simulink model "updated_target_driver_2026_withVariants_MPC_andwlqp2"  (R2024b)
settings: Solver=FixedStepDiscrete  StartTime=0.0  StopTime=running_time  FixedStep=dt_s  RelTol=1e-3
values from neighbouring files (symbols this model uses):
  A = gamma_2*gamma_3*Thrust_desired    [force2voltage.m]
  a2_lb = -0.25    [target_driver_setup_2022_Ctrl_V_2_4.m]    (also in target_driver_setup_2022_Ctrl_V_2_4_geometric.m; target_driver_setup_mpc_12msdelay.m; target_driver_setup_mpc_andWLQP.m)
  a2_openloop = -0    (= 0)    [target_driver_setup_2022_Ctrl_V_2_4.m]    (also in target_driver_setup_2022_Ctrl_V_2_4_geometric.m; target_driver_setup_mpc_12msdelay.m; target_driver_setup_mpc_andWLQP.m)
  a2_ub = 0.25    [target_driver_setup_2022_Ctrl_V_2_4.m]    (also in target_driver_setup_2022_Ctrl_V_2_4_geometric.m; target_driver_setup_mpc_12msdelay.m; target_driver_setup_mpc_andWLQP.m)
  att_s = 500    [target_driver_setup_2022_Ctrl_V_2_4.m]    (also in target_driver_setup_2022_Ctrl_V_2_4_geometric.m; target_driver_setup_mpc_12msdelay.m; target_driver_setup_mpc_andWLQP.m)
  c_vertical = 0.70e-3    (= 0.0007)    [target_driver_setup_mpc_andWLQP.m]
  closedloop_flag = 1    [target_driver_setup_2022_Ctrl_V_2_4.m]    (also in target_driver_setup_2022_Ctrl_V_2_4_geometric.m = 0; target_driver_setup_mpc_12msdelay.m = 0; target_driver_setup_mpc_andWLQP.m = 0)
  delay = delay-vicon_sample_cycle/2    [target_driver_setup_2022_Ctrl_V_2_4.m]    (also in target_driver_setup_2022_Ctrl_V_2_4_geometric.m; target_driver_setup_mpc_12msdelay.m; target_driver_setup_mpc_andWLQP.m)
  drv_amp = abs((vleft_p2p-vright_p2p))/2+min(vleft_p2p,vright_p2p)    [Wing_traj_to_Voltage.m]    (also in force2voltage.m; target_driver_setup_2022_Ctrl_V_2_4.m = 300; target_driver_setup_2022_Ctrl_V_2_4_geometric.m = 110; target_driver_setup_mpc_12msdelay.m = 150)
  drv_bias = max_drv_bias    (= 300)    [target_driver_setup_2022_Ctrl_V_2_4.m]    (also in target_driver_setup_2022_Ctrl_V_2_4_geometric.m = 200; target_driver_setup_mpc_12msdelay.m = 200; target_driver_setup_mpc_andWLQP.m = 200)
  drv_pitch_left = vleft_pitch    [Wing_traj_to_Voltage.m]    (also in force2voltage.m = 0; target_driver_setup_2022_Ctrl_V_2_4.m = 0; target_driver_setup_2022_Ctrl_V_2_4_geometric.m = 9.05; target_driver_setup_mpc_12msdelay.m = 9.05)
  drv_pitch_right = vright_pitch    [Wing_traj_to_Voltage.m]    (also in force2voltage.m = 0; target_driver_setup_2022_Ctrl_V_2_4.m = 0; target_driver_setup_2022_Ctrl_V_2_4_geometric.m = 9.05; target_driver_setup_mpc_12msdelay.m = 9.05)
  drv_roll = (vleft_p2p-vright_p2p)/4    [Wing_traj_to_Voltage.m]    (also in force2voltage.m; target_driver_setup_2022_Ctrl_V_2_4.m = 0; target_driver_setup_2022_Ctrl_V_2_4_geometric.m = -0.001; target_driver_setup_mpc_12msdelay.m = -0.001)
  dt_s = 1e-3    (= 0.001)    [target_driver_setup_2022_Ctrl_V_2_4.m]    (also in target_driver_setup_2022_Ctrl_V_2_4_geometric.m = 0.0002; target_driver_setup_mpc_12msdelay.m = 0.0002; target_driver_setup_mpc_andWLQP.m = 2.0e-4;1)
  f_fin = f    (= 180)    [target_driver_setup_2022_Ctrl_V_2_4.m]    (also in target_driver_setup_2022_Ctrl_V_2_4_geometric.m = 155; target_driver_setup_mpc_12msdelay.m = 155; target_driver_setup_mpc_andWLQP.m = 155)
  f_int = f    (= 180)    [target_driver_setup_2022_Ctrl_V_2_4.m]    (also in target_driver_setup_2022_Ctrl_V_2_4_geometric.m = 155; target_driver_setup_mpc_12msdelay.m = 155; target_driver_setup_mpc_andWLQP.m = 155)
  g = 9.8    [target_driver_setup_2022_Ctrl_V_2_4.m]    (also in target_driver_setup_2022_Ctrl_V_2_4_geometric.m; target_driver_setup_mpc_12msdelay.m; target_driver_setup_mpc_andWLQP.m = 9.81; test_full_attitude_mpc.m = 9.81)
  I_moment = eye(3)    [target_driver_exec_2022_Ctrl_V_2_4.m]    (also in target_driver_setup_2022_Ctrl_V_2_4.m; target_driver_setup_2022_Ctrl_V_2_4_geometric.m; target_driver_setup_mpc_12msdelay.m; target_driver_setup_mpc_andWLQP.m)
  k_tau_vec = [k_tau_roll;k_tau_pitch]    [target_driver_setup_2022_Ctrl_V_2_4_geometric.m]    (also in target_driver_setup_mpc_12msdelay.m; target_driver_setup_mpc_andWLQP.m)
  m = t <= t_zoom    [plot_roll_torque_cmd_vs_actual.m]    (also in plot_roll_torque_cmd_vs_actual_flightlog.m = t >= t0 & t <= t1; target_driver_setup_2022_Ctrl_V_2_4.m = 0.000124; target_driver_setup_2022_Ctrl_V_2_4_geometric.m = 8.5655e-05; target_driver_setup_mpc_12msdelay.m = 8.5655e-05)
  params_vec = [params_opt.delta_1, params_opt.delta_2, params_opt.delta_3,      params_opt.gamma_1, params_opt.gamma_2_1, params_opt.gamma_3,      params_opt.eta, params_opt.nu, params_opt.mu]'    [force2voltage_tuningSandbox.m]    (also in target_driver_setup_2022_Ctrl_V_2_4.m = [params_opt.delta_1, params_opt.delta_2, params_opt.delta_3,; target_driver_setup_2022_Ctrl_V_2_4_geometric.m = [params_opt.delta_1, params_opt.delta_2, params_opt.delta_3,; target_driver_setup_mpc_12msdelay.m = [params_opt.delta_1, params_opt.delta_2, params_opt.delta_3,; target_driver_setup_mpc_andWLQP.m = [params_opt.delta_1, params_opt.delta_2, params_opt.delta_3,)
  phase = 0    [target_driver_setup_2022_Ctrl_V_2_4.m]    (also in target_driver_setup_2022_Ctrl_V_2_4_geometric.m; target_driver_setup_mpc_12msdelay.m; target_driver_setup_mpc_andWLQP.m)
  popts_flattened = popts.popts    [target_driver_setup_mpc_andWLQP.m]
  roll_offset_angle = 0    [target_driver_setup_2022_Ctrl_V_2_4.m]    (also in target_driver_setup_2022_Ctrl_V_2_4_geometric.m; target_driver_setup_mpc_12msdelay.m; target_driver_setup_mpc_andWLQP.m)
  running_time = start_delay+total_T    (= 9)    [target_driver_setup_2022_Ctrl_V_2_4.m]    (also in target_driver_setup_2022_Ctrl_V_2_4_geometric.m = 10; target_driver_setup_mpc_12msdelay.m = 0.5; target_driver_setup_mpc_andWLQP.m = 10)
  running_time_control = start_delay_control+total_T+0.0    (= 7.1)    [target_driver_setup_2022_Ctrl_V_2_4.m]    (also in target_driver_setup_2022_Ctrl_V_2_4_geometric.m = 10; target_driver_setup_mpc_12msdelay.m = 0.5; target_driver_setup_mpc_andWLQP.m = 10)
  sampling_f = 10000    [target_driver_setup_2022_Ctrl_V_2_4.m]    (also in target_driver_setup_2022_Ctrl_V_2_4_geometric.m = 5000; target_driver_setup_mpc_12msdelay.m = 5000; target_driver_setup_mpc_andWLQP.m = 1/dt_s)
  start_delay = 2.0    (= 2)    [target_driver_setup_2022_Ctrl_V_2_4.m]    (also in target_driver_setup_2022_Ctrl_V_2_4_geometric.m = 0; target_driver_setup_mpc_12msdelay.m = 0; target_driver_setup_mpc_andWLQP.m = 0)
  start_delay_control = start_delay + ramp_delay    (= 0.1)    [target_driver_setup_2022_Ctrl_V_2_4.m]    (also in target_driver_setup_2022_Ctrl_V_2_4_geometric.m = 0; target_driver_setup_mpc_12msdelay.m = 0; target_driver_setup_mpc_andWLQP.m = 0)
  T = 1    [target_driver_setup_2022_Ctrl_V_2_4.m]    (also in target_driver_setup_2022_Ctrl_V_2_4_geometric.m = 10; target_driver_setup_mpc_12msdelay.m = 0.5; target_driver_setup_mpc_andWLQP.m = 10; test_full_attitude_mpc.m = T0 + nu(1))
  weights_vec = [ws; wds; wpr_xy;wpr_z; wpf; wvr_xy; wvr_z ... (first row only)    [target_driver_setup_2022_Ctrl_V_2_4_geometric.m]    (also in target_driver_setup_mpc_12msdelay.m; target_driver_setup_mpc_andWLQP.m)
undefined symbols (not defined in the file or in its folder): Com1, ctrl_Ts, DiscIntNeverNeededParam, dspblkCoreblockFVToolHelper, gcbh, left_mapping, left_mapping_F_to_Phi, lp_den, lp_num, none, right_mapping, right_mapping_F_to_Phi
libraries: simulink x17, xpcseriallib x2, cstblocks x1, xpcnilib x1, xpcutilitieslib x1
(part 1 of 4)
settings Model: PacingRate=0.020000  Creator=franklinho  LastModifiedBy=franklinho
settings DebuggingCC: SignalInfNanChecking=error  UnderSpecifiedDimensionMsg=warning

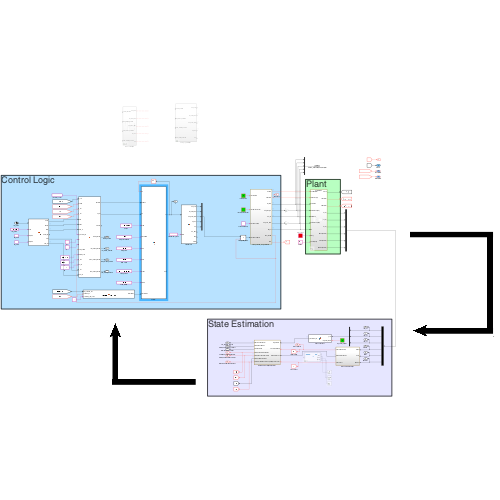
[thumbnail: Simulink's stored preview of the top-level diagram]
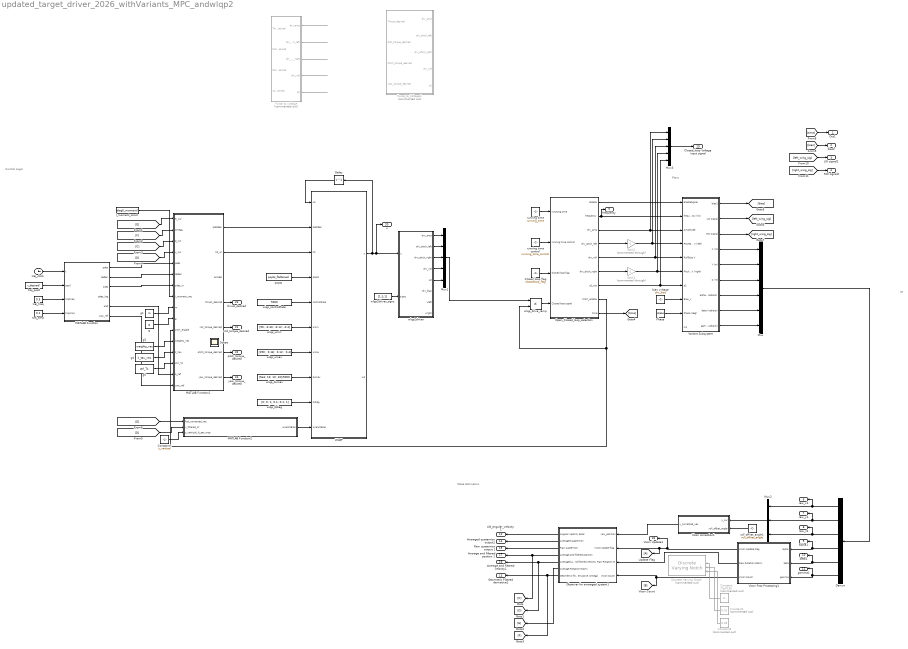
== system updated_target_driver_2026_withVariants_MPC_andwlqp2 ==
  note: te
  note: Plant
  note: State Estimation
  note: Control Logic
  Closed loop flag : Constant  Value=closedloop_flag
  Constant : Constant  Commented=on  Value=2*pi*155
  Constant1 : Constant  Commented=on  Value=0.01
  Constant2 : Constant  Commented=on  Value=0.05
  Constant3 : Constant  Value=c_vertical
  Delay : Delay  DelayLength=1  InitialCondition=[120; 0; 0; 0]
  Demux : Demux  Outputs=6
  Discrete Varying Notch : cstblocks/Linear Parameter Varying/Discrete Varying Notch  Commented=on  w0=973.894  Ts=2e-4
  Force to voltage : Subsystem  Commented=on  Variant=on
  Force_to_Voltage1 : Subsystem  Commented=on
  Gain2 : Gain  Commented=through  Gain=-1
  Gain3 : Gain  Commented=through  Gain=-1
  I_moment_const : Constant  Value=diag(I_moment)
  MATLAB Function : MATLAB Function  TreatAsAtomicUnit=on
  MATLAB Function1 : MATLAB Function  TreatAsAtomicUnit=on
  MATLAB Function2 : MATLAB Function  TreatAsAtomicUnit=on
  Mux : Mux  Inputs=6
  Mux1 : Mux  Inputs=5
  Mux2 : Mux  Inputs=3
  Mux3 : Mux  Inputs=5
  Observer for averaged system1 : Subsystem
  Open_Closed_loop_selection : Subsystem
  Phase : Constant  Value=phase
  Update Flag : Goto
  Variant Subsystem : Subsystem  Variant=on
  Vicon Post Processing1 : Subsystem
  Vicon correction1 : MATLAB Function  TreatAsAtomicUnit=on
  WLQP : MATLAB Function  TreatAsAtomicUnit=on
  bias voltage : Constant  Value=drv_bias
  g : Constant  Value=g
  g1 : Constant  Value=m
  g3 : Constant  Value=weights_vec
  g4 : Constant  Value=k_tau_vec
  g5 : Constant  Value=ctrl_Ts
  popts : Constant  Value=popts_flattened
  roll_offset_angle1 : Constant  Value=roll_offset_angle  SampleTime=-1
  running time : Constant  Value=running_time  SampleTime=-1
  running time control : Constant  Value=running_time_control  SampleTime=-1
  traj_amp : Constant  Value=0.1
  traj_clock : Clock
  traj_freq : Constant  Value=0.5
  traj_pos0 : Constant  Value=r_desired'
  wlqp2driver : MATLAB Function  TreatAsAtomicUnit=on
  wlqp2driver_signs : Constant  Value=[1;1;1]
  wlqp_Qdiag : Constant  Value=[0; 0; 1; 0.1; 0.1; 1]
  wlqp_controlRate : Constant  Value=5000
  wlqp_drive_ramp : Product
  wlqp_dumax : Constant  Value=[5e3; 10; 10; 10]/5000
  wlqp_umax : Constant  Value="[190;  0.18;  0.12;  0.4]"
  wlqp_umin : Constant  Value=[90; -0.40; -0.12; -0.4]
  Out1 : Outport
  bias2 : Outport  Port=2
  LW signal2 : Outport  Port=3
  RW signal2 : Outport  Port=4
  frequency : Outport  Port=5
  raw_x1 : Outport  Port=6
  raw_y1 : Outport  Port=7
  raw_z1 : Outport  Port=8
  alpha1 : Outport  Port=9
  beta1 : Outport  Port=10
  gamma1 : Outport  Port=11
  old_angular_velocity 1 : Outport  Port=12
  Geometric Filtered derivative1 : Outport  Port=13
  Averaged quaternion output1 : Outport  Port=14
  Raw quaternion output 1 : Outport  Port=15
  Average and filtered velocity1 : Outport  Port=16
  Average and filtered position 1 : Outport  Port=17
  Vicon Update1 : Outport  Port=18
  Closed_loop Voltage input signal : Outport  Port=19
  u : Outport  Port=20
  roll_torque_desired : Outport  Port=21
  pitch_torque_desired : Outport  Port=22
  thrust_desired : Outport  Port=23
  yaw_torque_desired : Outport  Port=24
  Scope : Scope
  wires:
  Observer for averaged system1/1("Angular velocity Euler ") -> old_angular_velocity 1/1
  Observer for averaged system1/5(Averaged and filtered velocity) -> [D], Average and filtered velocity1/1
  Observer for averaged system1/2(Averaged quaternion) -> Averaged quaternion output1/1
  roll_offset_angle1/1 -> Vicon correction1/2(roll_offset_angle)
  Observer for averaged system1/4("Average and filtered position ") -> Average and filtered position 1/1, [C]
  Observer for averaged system1/3(Raw quaternion) -> Raw quaternion output 1/1
  Vicon Post Processing1/1("Vicon Update Flag ") -> Vicon Update1/1, Update Flag/1, Observer for averaged system1/2(Vicon Update flag)
  Observer for averaged system1/7(Geometric filtered derivative (omega)) -> [F], Geometric Filtered derivative1/1
  Mux2/1 -> Vicon correction1/1(x_cur)
  Vicon Post Processing1/3("Vicon Count ") -> Observer for averaged system1/4(Vicon Count), [B]
  Vicon correction1/1(x_corrected_vec) -> Observer for averaged system1/1("raw_position ")
  Variant Subsystem/4(X (m)) -> Mux/1
  Variant Subsystem/5(Y (m)) -> Mux/2
  Variant Subsystem/6(Z (m)) -> Mux/3
  Variant Subsystem/7(alpha (radians)) -> Mux/4
  Variant Subsystem/8(beta (radians)) -> Mux/5
  Variant Subsystem/9(gamma (radians)) -> Mux/6
  Variant Subsystem/1(bias2) -> [bias]
  Variant Subsystem/2(LW signal) -> [left_wing_sig]
  Variant Subsystem/3(RW signal) -> [right_wing_sig]
  Mux/1 -> Demux/1
  Demux/1 -> raw_x1/1, Mux2/1
  Demux/3 -> raw_z1/1, Mux2/3
  Demux/2 -> raw_y1/1, Mux2/2
  Demux/4 -> alpha1/1, Vicon Post Processing1/1(alpha)
  Demux/5 -> beta1/1, Vicon Post Processing1/2(beta)
  Demux/6 -> gamma1/1, Vicon Post Processing1/3(gamma)
  running time control/1 -> Open_Closed_loop_selection/2("running time control ")
  Closed loop flag/1 -> Open_Closed_loop_selection/3(Closed loop flag)
  running time/1 -> Open_Closed_loop_selection/1(runnting time)
  Open_Closed_loop_selection/1("Enable ") -> Variant Subsystem/1(EnableSignal)
  Open_Closed_loop_selection/2(frequency) -> Variant Subsystem/2(frequency (hz)), frequency/1
  Open_Closed_loop_selection/3(drv_amp) -> Mux3/1, Variant Subsystem/3(Amplitude)
  Open_Closed_loop_selection/4("drv_pitch_left ") -> Gain2/1
  Open_Closed_loop_selection/6("drv_pitch_right ") -> Gain3/1
  Open_Closed_loop_selection/7(a2_out) -> Mux3/5, Variant Subsystem/7(a2)
  Open_Closed_loop_selection/9(time) -> [time]
  bias voltage/1 -> Variant Subsystem/8(Bias_v)
  Phase/1 -> Variant Subsystem/9(Phase (deg))
  Mux3/1 -> Closed_loop Voltage input signal/1
  [time] -> Out1/1
  [bias] -> bias2/1
  [left_wing_sig] -> LW signal2/1
  [right_wing_sig] -> RW signal2/1
  Open_Closed_loop_selection/5("drv_roll ") -> Mux3/3, Variant Subsystem/5(RollBias V)
  Vicon Post Processing1/2(Raw Rotation Matrix) -> Observer for averaged system1/3("Raw Rotation M ")
  Constant/1 -> Discrete Varying Notch/2
  Constant1/1 -> Discrete Varying Notch/3
  Constant2/1 -> Discrete Varying Notch/4
  Gain2/1 -> Mux3/2, Variant Subsystem/4(PitchBias V (left))
  Gain3/1 -> Mux3/4, Variant Subsystem/6(PitchBias V (right))
  g/1 -> MATLAB Function1/10(g)
  g1/1 -> MATLAB Function1/9(m)
  MATLAB Function/1(pdes) -> MATLAB Function1/5(pdes)
  MATLAB Function/2(dpdes) -> MATLAB Function1/6(dpdes)
  MATLAB Function/3(sdes) -> MATLAB Function1/7(sdes_in)
  [E] -> MATLAB Function1/1(R_cur)
  [F] -> MATLAB Function1/2(omega)
  Open_Closed_loop_selection/8(Cntrl_enable) -> wlqp_drive_ramp/2, MATLAB Function1/11(cntrl_enable)
  g3/1 -> MATLAB Function1/12(weights_vec)
  g4/1 -> MATLAB Function1/13(k_tau)
  g5/1 -> MATLAB Function1/14(ctrl_Ts)
  [C] -> MATLAB Function1/3(p_cur)
  [D] -> MATLAB Function1/4(v_cur)
  WLQP/1(u) -> u/1, wlqp2driver/1(u), Delay/1
  Delay/1 -> WLQP/1(u0)
  MATLAB Function1/2(h0_wl) -> WLQP/3(h0)
  MATLAB Function1/1(pdotdes) -> WLQP/2(pdotdes)
  Force to voltage/2(drv_pitch_left) -> ?
  Force to voltage/4(drv_roll) -> ?
  Force to voltage/5(a2) -> ?
  Force to voltage/3(drv_pitch_right) -> ?
  Force to voltage/1(drv_amp) -> ?
  wlqp2driver/1(drv_amp) -> Mux1/1
  wlqp2driver/2(drv_pitch_left) -> Mux1/2
  wlqp2driver/3(drv_pitch_right) -> Mux1/3
  wlqp2driver/4(drv_roll) -> Mux1/4
  wlqp2driver/5(a2) -> Mux1/5
  popts/1 -> WLQP/4(popts)
  traj_clock/1 -> MATLAB Function/1(t)
  traj_pos0/1 -> MATLAB Function/2(pos0)
  traj_freq/1 -> MATLAB Function/3(trajFreq)
  traj_amp/1 -> MATLAB Function/4(trajAmp)
  I_moment_const/1 -> MATLAB Function1/8(I_moment_vec)
  wlqp_controlRate/1 -> WLQP/5(controlRate)
  wlqp_umin/1 -> WLQP/6(umin)
  wlqp_umax/1 -> WLQP/7(umax)
  wlqp_dumax/1 -> WLQP/8(dumax)
  wlqp_Qdiag/1 -> WLQP/9(Qdiag)
  MATLAB Function1/5(roll_torque_desired) -> roll_torque_desired/1
  MATLAB Function1/6(pitch_torque_desired) -> pitch_torque_desired/1
  wlqp2driver_signs/1 -> wlqp2driver/2(signs)
  MATLAB Function1/4(thrust_desired) -> thrust_desired/1
  Mux1/1 -> wlqp_drive_ramp/1
  wlqp_drive_ramp/1 -> Open_Closed_loop_selection/4(Closed loop signal)
  MATLAB Function/5(aref) -> MATLAB Function1/15(a_ref)
  MATLAB Function1/7(yaw_torque_desired) -> yaw_torque_desired/1
  Observer for averaged system1/6(Average Rotation Matrix) -> [E]
  MATLAB Function2/1(wrenchBias) -> WLQP/10(wrenchBias)
  [D] -> MATLAB Function2/2(v_filtered_W)
  Constant3/1 -> MATLAB Function2/3(c_vertical_N_per_mps)
  [E] -> MATLAB Function2/1(Rot_corrected_vec)
  MATLAB Function/6(yaw_ref) -> MATLAB Function1/16(yaw_ref)

== system updated_target_driver_2026_withVariants_MPC_andwlqp2/Force to voltage ==
  note: 1) Add Subsystem or Model blocks as valid variant choices.
      | 2) You cannot connect blocks at this level. At simulation, connectivity is automatically
      | determined, based on the active variant and port name matching.
  "Thrust_desired " : Inport
  Roll_torque_desired : Inport  Port=2
  Pitch_torque_desired : Inport  Port=3
  Yaw_torque_desired : Inport  Port=4
  Control Mode : Subsystem  VariantControl=replay_mode==1
  Replay Mode : Subsystem  VariantControl=replay_mode==2
  drv_amp : Outport
  drv_pitch_left : Outport  Port=2
  drv_pitch_right : Outport  Port=3
  drv_roll : Outport  Port=4
  a2 : Outport  Port=5

== system updated_target_driver_2026_withVariants_MPC_andwlqp2/Force_to_Voltage1 ==
  note: Mapping from desired Thrust/Torque to Wing traj to Voltage mapping
      |
      | Patrick Hyun 2021 Apr
  note: a2: second-harmonic coefficient
      | Franklin Ho Jun 2026
  "Thrust_desired " : Inport
  Roll_torque_desired : Inport  Port=2
  Pitch_torque_desired : Inport  Port=3
  Yaw_torque_desired : Inport  Port=4
  A : Constant  Commented=on  Value=A
  Desired_Force_to_Voltage : MATLAB Function  TreatAsAtomicUnit=on
  "Force to Trajectory " : MATLAB Function  Commented=on  TreatAsAtomicUnit=on
  Saturation : Saturate  UpperLimit=a2_ub  LowerLimit=a2_lb
  "Trajectory to Voltage Input " : MATLAB Function  Commented=on  TreatAsAtomicUnit=on
  left_mapping : Constant  Commented=on  Value=left_mapping
  left_mapping_F_to_Phi : Constant  Commented=on  Value=left_mapping_F_to_Phi
  params_vec : Constant  Value=params_vec
  right_mapping1 : Constant  Commented=on  Value=right_mapping
  right_mapping_F_to_Phi : Constant  Commented=on  Value=right_mapping_F_to_Phi
  drv_amp : Outport
  drv_pitch_left : Outport  Port=2
  drv_pitch_right : Outport  Port=3
  drv_roll : Outport  Port=4
  a2 : Outport  Port=5
  wires:
  left_mapping/1 -> "Trajectory to Voltage Input "/4(left_mapping)
  right_mapping1/1 -> "Trajectory to Voltage Input "/5(right_mapping)
  A/1 -> "Force to Trajectory "/6(A)
  "Force to Trajectory "/1(Phi_left_p2p_desired) -> "Trajectory to Voltage Input "/1(Phi_left_p2p_command)
  "Force to Trajectory "/2(Phi_right_p2p_desired) -> "Trajectory to Voltage Input "/2(Phi_right_p2p_command)
  "Force to Trajectory "/3(Phi_pitch_desired) -> "Trajectory to Voltage Input "/3(Phi_pitch_command)
  left_mapping_F_to_Phi/1 -> "Force to Trajectory "/4(left_mapping_F_to_Phi)
  right_mapping_F_to_Phi/1 -> "Force to Trajectory "/5(right_mapping_F_to_Phi)
  Desired_Force_to_Voltage/4(drv_pitch_right) -> drv_pitch_right/1
  Desired_Force_to_Voltage/3(drv_pitch_left) -> drv_pitch_left/1
  Desired_Force_to_Voltage/2(drv_roll) -> drv_roll/1
  Desired_Force_to_Voltage/1(drv_amp) -> drv_amp/1
  "Thrust_desired "/1 -> Desired_Force_to_Voltage/1(Thrust_desired)
  Pitch_torque_desired/1 -> Desired_Force_to_Voltage/3(Pitch_torque_desired)
  Yaw_torque_desired/1 -> Desired_Force_to_Voltage/4(Yaw_torque_desired)
  params_vec/1 -> Desired_Force_to_Voltage/5(params_vec)
  Desired_Force_to_Voltage/5(a2_coeff) -> Saturation/1
  Saturation/1 -> a2/1
  Roll_torque_desired/1 -> Desired_Force_to_Voltage/2(Roll_torque_desired)

== system updated_target_driver_2026_withVariants_MPC_andwlqp2/Observer for averaged system1 ==
  note: Observer for averaged system using geoemtric average
      | Includes the Euler derivatives to compute the angular velocity (probably not used for control)
      | Includes the geometric average and the first order derivative in Riemannian metric SO(3)
      |
      | Patrick 2021 Mar
  "raw_position " : Inport
  Vicon Update flag : Inport  Port=2
  "Raw Rotation M " : Inport  Port=3
  Vicon Count : Inport  Port=4
  Attitude Observer : Subsystem
  "Euler derivative & filtered angular velocity " : Subsystem
  Position Observer : Subsystem
  Terminator : Terminator
  "Angular velocity Euler " : Outport
  Averaged quaternion : Outport  Port=2
  Raw quaternion : Outport  Port=3
  "Average and filtered position " : Outport  Port=4
  Averaged and filtered velocity : Outport  Port=5
  Average Rotation Matrix : Outport  Port=6
  Geometric filtered derivative (omega) : Outport  Port=7
  wires:
  "Raw Rotation M "/1 -> "Euler derivative & filtered angular velocity "/1("Rotation matrix "), Attitude Observer/2(Raw Rotation)
  Vicon Count/1 -> Attitude Observer/3(Vicon Count), Position Observer/3(Vicon Count)
  "raw_position "/1 -> Position Observer/1("raw_position ")
  Position Observer/1(Average and filtered position) -> "Average and filtered position "/1
  Position Observer/2(Averaged and filtered velocity) -> Averaged and filtered velocity/1
  "Euler derivative & filtered angular velocity "/1(Angular velocity_Euler) -> "Angular velocity Euler "/1
  Vicon Update flag/1 -> Attitude Observer/1(Vicon Update flag), Position Observer/2(vicon Update)
  Attitude Observer/1("Averaged quaternion ") -> Averaged quaternion/1
  Attitude Observer/2(Average Rotation Matrix) -> Average Rotation Matrix/1
  Attitude Observer/3(Raw quaternion) -> Raw quaternion/1
  Attitude Observer/4(Geometric filtered derivative) -> Geometric filtered derivative (omega)/1
  "Euler derivative & filtered angular velocity "/2(Frob_norm error) -> Terminator/1

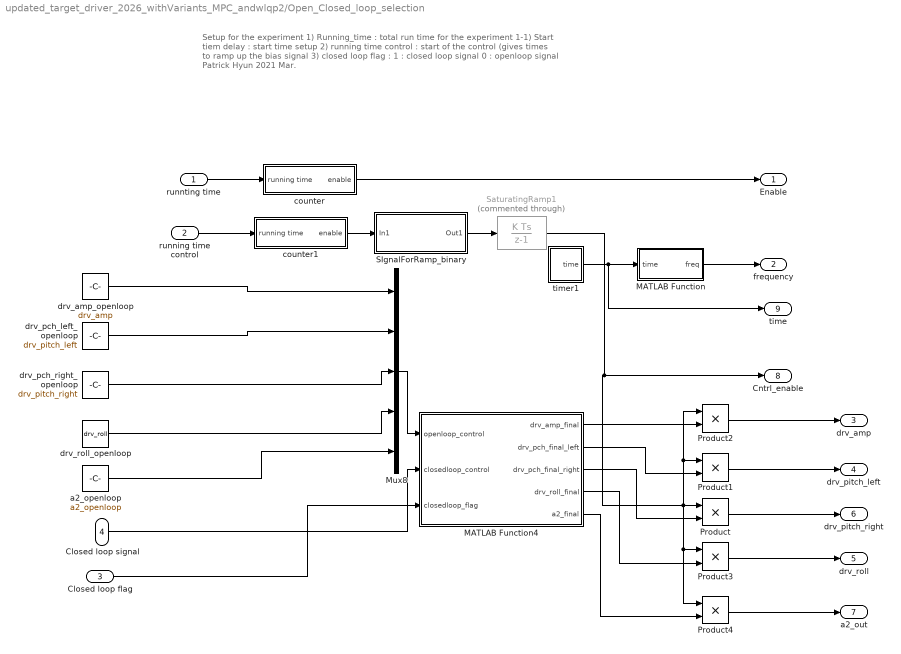
== system updated_target_driver_2026_withVariants_MPC_andwlqp2/Open_Closed_loop_selection ==
  note: Setup for the experiment
      |
      | 1) Running_time : total run time for the experiment
      | 1-1) Start tiem delay : start time setup
      | 2) running time control : start of the control (gives times to ramp up the bias signal
      | 3) closed loop flag : 1 : closed loop signal 0 : openloop signal
      |
      | Patrick Hyun 2021 Mar.
  runnting time : Inport
  "running time control " : Inport  Port=2
  Closed loop flag : Inport  Port=3
  Closed loop signal : Inport  Port=4
  MATLAB Function : MATLAB Function  TreatAsAtomicUnit=on
  MATLAB Function4 : MATLAB Function  TreatAsAtomicUnit=on
  Mux8 : Mux  Inputs=5
  Product{,1..4} (5 alike) : Product  RndMeth=Zero
  SIgnalForRamp_binary : Subsystem
  SaturatingRamp1 : DiscreteIntegrator  Commented=through  gainval=2.5  SampleTime=-1  LimitOutput=on  UpperSaturationLimit=1  LowerSaturationLimit=0  ICPrevOutput=DiscIntNeverNeededParam  ICPrevScaledInput=DiscIntNeverNeededParam
  a2_openloop : Constant  Value=a2_openloop
  counter : Subsystem
  counter1 : Subsystem
  "drv_amp_openloop " : Constant  Value=drv_amp
  drv_pch_left_openloop : Constant  Value=drv_pitch_left
  drv_pch_right_openloop : Constant  Value=drv_pitch_right
  "drv_roll_openloop " : Constant  Value=drv_roll
  timer1 : Subsystem
  "Enable " : Outport
  frequency : Outport  Port=2
  drv_amp : Outport  Port=3
  "drv_pitch_left " : Outport  Port=4
  "drv_roll " : Outport  Port=5
  "drv_pitch_right " : Outport  Port=6
  a2_out : Outport  Port=7
  Cntrl_enable : Outport  Port=8
  time : Outport  Port=9
  wires:
  runnting time/1 -> counter/1(running time)
  timer1/1(time) -> time/1, MATLAB Function/1(time)
  MATLAB Function/1(freq) -> frequency/1
  SIgnalForRamp_binary/1(Out1) -> SaturatingRamp1/1
  "drv_amp_openloop "/1 -> Mux8/1
  Product1/1 -> "drv_pitch_left "/1
  counter1/1(enable) -> SIgnalForRamp_binary/1(In1)
  "running time control "/1 -> counter1/1(running time)
  Product3/1 -> "drv_roll "/1
  Closed loop flag/1 -> MATLAB Function4/3(closedloop_flag)
  MATLAB Function4/4(drv_roll_final) -> Product3/2
  Mux8/1 -> MATLAB Function4/1(openloop_control)
  MATLAB Function4/2(drv_pch_final_left) -> Product1/2
  Product2/1 -> drv_amp/1
  MATLAB Function4/1(drv_amp_final) -> Product2/2
  drv_pch_left_openloop/1 -> Mux8/2
  MATLAB Function4/3(drv_pch_final_right) -> Product/2
  Product/1 -> "drv_pitch_right "/1
  counter/1(enable) -> "Enable "/1
  Closed loop signal/1 -> MATLAB Function4/2(closedloop_control)
  "drv_roll_openloop "/1 -> Mux8/4
  drv_pch_right_openloop/1 -> Mux8/3
  Product4/1 -> a2_out/1
  MATLAB Function4/5(a2_final) -> Product4/2
  a2_openloop/1 -> Mux8/5
  SaturatingRamp1/1 -> Product4/1, Product3/1, Product2/1, Product1/1, Product/1, Cntrl_enable/1

== system updated_target_driver_2026_withVariants_MPC_andwlqp2/Variant Subsystem ==
  note: 1) Add Subsystem or Model blocks as valid variant choices.
      | 2) You cannot connect blocks at this level. At simulation, connectivity is automatically
      | determined, based on the active variant and port name matching.
  EnableSignal : Inport
  frequency (hz) : Inport  Port=2
  Amplitude : Inport  Port=3
  PitchBias V (left) : Inport  Port=4
  RollBias V : Inport  Port=5
  PitchBias V (right) : Inport  Port=6
  a2 : Inport  Port=7
  Bias_v : Inport  Port=8
  Phase (deg) : Inport  Port=9
  In1 : Inport  Port=10
  Experimental : Subsystem  VariantControl=Plant==1
  Simulation : Subsystem  VariantControl=Plant==2
  bias2 : Outport
  LW signal : Outport  Port=2
  RW signal : Outport  Port=3
  X (m) : Outport  Port=4
  Y (m) : Outport  Port=5
  Z (m) : Outport  Port=6
  alpha (radians) : Outport  Port=7
  beta (radians) : Outport  Port=8
  gamma (radians) : Outport  Port=9

== system updated_target_driver_2026_withVariants_MPC_andwlqp2/Vicon Post Processing1 ==
  note: Process Vicon data
      |
      | 1) Generate Raw rotation matrix
      | 2) Flag the update of new vicon data
      | 3) Count the number of samples before new update
      |
      | By Patrick 2021 Mar
  alpha : Inport
  beta : Inport  Port=2
  gamma : Inport  Port=3
  Raw rotation matrix : Subsystem
  Vicon Validity check : Subsystem
  Vicon correction : MATLAB Function  TreatAsAtomicUnit=on
  roll_offset_angle : Constant  Value=roll_offset_angle  SampleTime=-1
  "Vicon Update Flag " : Outport
  Raw Rotation Matrix : Outport  Port=2
  "Vicon Count " : Outport  Port=3
  wires:
  Vicon Validity check/2(Vicon Count) -> "Vicon Count "/1
  beta/1 -> Raw rotation matrix/2(beta)
  gamma/1 -> Raw rotation matrix/3(gamma)
  alpha/1 -> Raw rotation matrix/1(alpha)
  Vicon Validity check/1("Vicon Update flag ") -> "Vicon Update Flag "/1
  roll_offset_angle/1 -> Vicon correction/2(roll_offset_angle)
  Raw rotation matrix/1(R) -> Vicon correction/1(R_cur)
  Vicon correction/1(Rot_corrected_vec) -> Raw Rotation Matrix/1, Vicon Validity check/1("Rotation Matrix ")

== system updated_target_driver_2026_withVariants_MPC_andwlqp2/Force to voltage/Control Mode ==
  "Thrust_desired " : Inport
  Roll_torque_desired : Inport  Port=2
  Pitch_torque_desired : Inport  Port=3
  Yaw_torque_desired : Inport  Port=4
  Desired_Force_to_Voltage : MATLAB Function  TreatAsAtomicUnit=on
  Force_to_Voltage1 : Subsystem  Commented=on
  Saturation : Saturate  UpperLimit=a2_ub  LowerLimit=a2_lb
  params_vec : Constant  Value=params_vec
  drv_amp : Outport
  drv_pitch_left : Outport  Port=2
  drv_pitch_right : Outport  Port=3
  drv_roll : Outport  Port=4
  a2 : Outport  Port=5
  wires:
  Desired_Force_to_Voltage/5(a2_coeff) -> Saturation/1
  Yaw_torque_desired/1 -> Desired_Force_to_Voltage/4(Yaw_torque_desired)
  Roll_torque_desired/1 -> Desired_Force_to_Voltage/2(Roll_torque_desired)
  Desired_Force_to_Voltage/1(drv_amp) -> drv_amp/1
  "Thrust_desired "/1 -> Desired_Force_to_Voltage/1(Thrust_desired)
  Desired_Force_to_Voltage/3(drv_pitch_left) -> drv_pitch_left/1
  Pitch_torque_desired/1 -> Desired_Force_to_Voltage/3(Pitch_torque_desired)
  params_vec/1 -> Desired_Force_to_Voltage/5(params_vec)
  Desired_Force_to_Voltage/4(drv_pitch_right) -> drv_pitch_right/1
  Desired_Force_to_Voltage/2(drv_roll) -> drv_roll/1
  Saturation/1 -> a2/1

== system updated_target_driver_2026_withVariants_MPC_andwlqp2/Force to voltage/Replay Mode ==
  "Thrust_desired " : Inport
  Roll_torque_desired : Inport  Port=2
  Pitch_torque_desired : Inport  Port=3
  Yaw_torque_desired : Inport  Port=4
  Demux4 : Demux
  Force_to_Voltage1 : Subsystem
  Replay commands : FromWorkspace  VariableName=robobee_load_replay_data(replay_log_file,'commands')  Interpolate=off  OutputAfterFinalValue=Holding final value
  Saturation : Saturate  UpperLimit=a2_ub  LowerLimit=a2_lb
  Term_{1..4} (4 alike) : Terminator
  drv_amp : Outport
  drv_pitch_left : Outport  Port=2
  drv_pitch_right : Outport  Port=3
  drv_roll : Outport  Port=4
  a2 : Outport  Port=5
  wires:
  Saturation/1 -> a2/1
  Force_to_Voltage1/5(a2) -> Saturation/1
  Force_to_Voltage1/4(drv_roll) -> drv_pitch_right/1
  Force_to_Voltage1/2(drv_pitch_left) -> drv_roll/1
  Force_to_Voltage1/3(drv_pitch_right) -> drv_pitch_left/1
  Force_to_Voltage1/1(drv_amp) -> drv_amp/1
  Replay commands/1 -> Demux4/1
  Demux4/1 -> Force_to_Voltage1/1("Thrust_desired ")
  Demux4/2 -> Force_to_Voltage1/2(Roll_torque_desired)
  Demux4/3 -> Force_to_Voltage1/3(Pitch_torque_desired)
  Demux4/4 -> Force_to_Voltage1/4(Yaw_torque_desired)
  "Thrust_desired "/1 -> Term_1/1
  Roll_torque_desired/1 -> Term_2/1
  Pitch_torque_desired/1 -> Term_3/1
  Yaw_torque_desired/1 -> Term_4/1

== system updated_target_driver_2026_withVariants_MPC_andwlqp2/Observer for averaged system1/Attitude Observer ==
  note: Attitude averaging and filtering using geometric average in Riemannian metric SO(3)
      |
      | Patrick 2021 Mar
  Vicon Update flag : Inport
  Raw Rotation : Inport  Port=2
  Vicon Count : Inport  Port=3
  Geometric Averaging Rotation Matix : Subsystem
  Geometric derivative in SO(3) : Subsystem
  "Averaged quaternion " : Outport
  Average Rotation Matrix : Outport  Port=2
  Raw quaternion : Outport  Port=3
  Geometric filtered derivative : Outport  Port=4
  wires:
  Vicon Count/1 -> Geometric derivative in SO(3)/2(Vicon Count)
  Raw Rotation/1 -> Geometric Averaging Rotation Matix/2(Current Rotation)
  Vicon Update flag/1 -> Geometric derivative in SO(3)/4("Vicon Update Flag "), Geometric Averaging Rotation Matix/1(Vicon Update flag)
  Geometric Averaging Rotation Matix/4(Previous Averaged Rotation Matrix) -> Geometric derivative in SO(3)/1(Previous Averaged Rotation M)
  Geometric derivative in SO(3)/1(Filtered Geometric derivative in SO(3)) -> Geometric filtered derivative/1
  Geometric Averaging Rotation Matix/3("Raw quaternion output ") -> Raw quaternion/1
  Geometric Averaging Rotation Matix/1(Averaged quaternion output) -> "Averaged quaternion "/1
  Geometric Averaging Rotation Matix/2("Averaged Rotation Matrix ") -> Average Rotation Matrix/1, Geometric derivative in SO(3)/3(Current Averaged Rotation M)

== system updated_target_driver_2026_withVariants_MPC_andwlqp2/Observer for averaged system1/Euler derivative & filtered angular velocity  ==
  note: The skew symmetric structure is corrected from
      | the old angular velocity calculation.
      | Note from Patrick 2021 Mar
  "Rotation matrix " : Inport
  Angular velocity : MATLAB Function  TreatAsAtomicUnit=on
  Demux : Demux  Outputs=3
  Mux : Mux  Inputs=3
  filtered derivative : Subsystem
  Angular velocity_Euler : Outport
  Frob_norm error : Outport  Port=2
  wires:
  Demux/2 -> Mux/2
  Demux/3 -> Mux/3
  Mux/1 -> Angular velocity_Euler/1
  filtered derivative/1(Out1) -> Angular velocity/2(Rdot)
  Angular velocity/1(w) -> Demux/1
  Demux/1 -> Mux/1
  Angular velocity/2(Frob_error) -> Frob_norm error/1
  "Rotation matrix "/1 -> Angular velocity/1(R), filtered derivative/1(In1)

== system updated_target_driver_2026_withVariants_MPC_andwlqp2/Observer for averaged system1/Position Observer ==
  "raw_position " : Inport
  vicon Update : Inport  Port=2
  Vicon Count : Inport  Port=3
  "Averaging position & velocity " : MATLAB Function  TreatAsAtomicUnit=on
  Constant : Constant  Value=sampling_f
  Delay10 : Delay  DelayLength=delay(2)  InitialCondition=0
  Delay11 : Delay  DelayLength=delay(3)  InitialCondition=0
  Delay14 : Delay  DelayLength=delay(4)  InitialCondition=0
  LowPassFilter1 : Subsystem
  LowPassFilter2 : Subsystem
  previous position : Delay  DelayLength=1  InitialCondition=0
  previous velocity : Delay  DelayLength=1  InitialCondition=0
  Average and filtered position : Outport
  Averaged and filtered velocity : Outport  Port=2
  wires:
  previous velocity/1 -> "Averaging position & velocity "/8(vout_prev)
  "Averaging position & velocity "/2(vout) -> previous velocity/1, LowPassFilter2/1(In1)
  previous position/1 -> "Averaging position & velocity "/7(rout_prev)
  "raw_position "/1 -> "Averaging position & velocity "/4(r_cur), Delay14/1, Delay11/1, Delay10/1
  Delay14/1 -> "Averaging position & velocity "/3(r_prev3)
  Delay11/1 -> "Averaging position & velocity "/2(r_prev2)
  Delay10/1 -> "Averaging position & velocity "/1(r_prev)
  LowPassFilter2/1(Out1) -> Averaged and filtered velocity/1
  "Averaging position & velocity "/1(rout) -> previous position/1, LowPassFilter1/1(In1)
  LowPassFilter1/1(Out1) -> Average and filtered position/1
  vicon Update/1 -> "Averaging position & velocity "/5(update)
  Vicon Count/1 -> "Averaging position & velocity "/6(count)
  Constant/1 -> "Averaging position & velocity "/9(sampling_f)

== system updated_target_driver_2026_withVariants_MPC_andwlqp2/Open_Closed_loop_selection/SIgnalForRamp_binary ==
  note: Should output 1 or -1,
      | so signal ramps UP to 1
      | or DOWN to 0.
  In1 : Inport
  Add : Sum  Inputs=+-
  Compare To Zero : simulink/Logic and Bit Operations/Compare To Zero  relop=>  OutDataTypeStr=uint8  ZeroCross=off
  Constant : Constant
  Data Type Conversion : DataTypeConversion  OutDataTypeStr=double  SaturateOnIntegerOverflow=off  RndMeth=Floor
  Gain : Gain  Gain=2
  Out1 : Outport
  wires:
  In1/1 -> Compare To Zero/1
  Compare To Zero/1 -> Data Type Conversion/1
  Gain/1 -> Add/1
  Constant/1 -> Add/2
  Add/1 -> Out1/1
  Data Type Conversion/1 -> Gain/1

== system updated_target_driver_2026_withVariants_MPC_andwlqp2/Open_Closed_loop_selection/counter ==
  running time : Inport
  Add : Sum  Inputs=+-
  Compare To Zero : simulink/Logic and Bit Operations/Compare To Zero  relop=<  OutDataTypeStr=uint8  ZeroCross=off
  Product2 : Product  RndMeth=Zero
  SaturatingRamp : DiscreteIntegrator  gainval=1  SampleTime=-1  UpperSaturationLimit=1  LowerSaturationLimit=0  ICPrevOutput=DiscIntNeverNeededParam  ICPrevScaledInput=DiscIntNeverNeededParam
  constant : Constant
  start delay compare : simulink/Logic and Bit Operations/Compare To Constant  relop=>  const=start_delay  OutDataTypeStr=uint8
  enable : Outport
  wires:
  SaturatingRamp/1 -> Add/1, start delay compare/1
  running time/1 -> Add/2
  Add/1 -> Compare To Zero/1
  start delay compare/1 -> Product2/1
  Compare To Zero/1 -> Product2/2
  Product2/1 -> enable/1
  constant/1 -> SaturatingRamp/1

== system updated_target_driver_2026_withVariants_MPC_andwlqp2/Open_Closed_loop_selection/counter1 ==
  running time : Inport
  Add : Sum  Inputs=+-
  Compare To Zero : simulink/Logic and Bit Operations/Compare To Zero  relop=<  OutDataTypeStr=uint8  ZeroCross=off
  Product2 : Product  RndMeth=Zero
  SaturatingRamp : DiscreteIntegrator  gainval=1  SampleTime=-1  UpperSaturationLimit=1  LowerSaturationLimit=0  ICPrevOutput=DiscIntNeverNeededParam  ICPrevScaledInput=DiscIntNeverNeededParam
  constant : Constant
  start control delay compare : simulink/Logic and Bit Operations/Compare To Constant  relop=>  const=start_delay_control  OutDataTypeStr=uint8
  enable : Outport
  wires:
  SaturatingRamp/1 -> Add/1, start control delay compare/1
  running time/1 -> Add/2
  Add/1 -> Compare To Zero/1
  start control delay compare/1 -> Product2/1
  Compare To Zero/1 -> Product2/2
  Product2/1 -> enable/1
  constant/1 -> SaturatingRamp/1

== system updated_target_driver_2026_withVariants_MPC_andwlqp2/Open_Closed_loop_selection/timer1 ==
  SaturatingRamp : DiscreteIntegrator  gainval=1  SampleTime=-1  UpperSaturationLimit=1  LowerSaturationLimit=0  ICPrevOutput=DiscIntNeverNeededParam  ICPrevScaledInput=DiscIntNeverNeededParam
  constant : Constant
  time : Outport
  wires:
  SaturatingRamp/1 -> time/1
  constant/1 -> SaturatingRamp/1

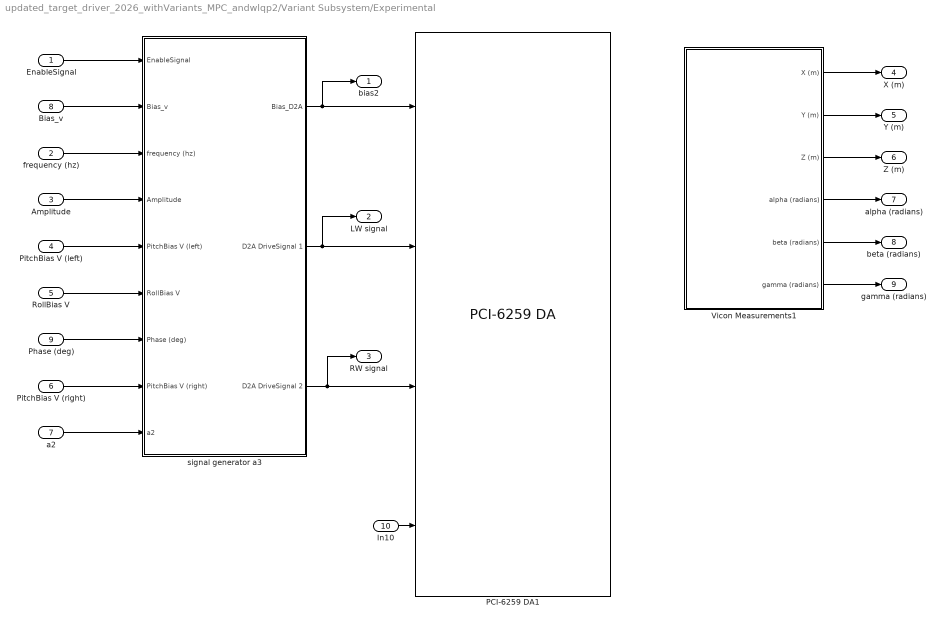
== system updated_target_driver_2026_withVariants_MPC_andwlqp2/Variant Subsystem/Experimental ==
  EnableSignal : Inport
  frequency (hz) : Inport  Port=2
  Amplitude : Inport  Port=3
  PitchBias V (left) : Inport  Port=4
  RollBias V : Inport  Port=5
  PitchBias V (right) : Inport  Port=6
  a2 : Inport  Port=7
  Bias_v : Inport  Port=8
  Phase (deg) : Inport  Port=9
  In10 : Inport  Port=10
  PCI-6259 DA1 : xpcnilib/D//A/M Series/PCI-6259 DA  channel=[1:4]  range=[10,5, 10, 10]  reset=[1 1 1 1]  initValue=[0 0 0 0]  sampletime=-1  slot=-1
      settings: SourceProductName=Simulink Real-Time
  Vicon Measurements1 : Subsystem
  signal generator a3 : Subsystem
  bias2 : Outport
  LW signal : Outport  Port=2
  RW signal : Outport  Port=3
  X (m) : Outport  Port=4
  Y (m) : Outport  Port=5
  Z (m) : Outport  Port=6
  alpha (radians) : Outport  Port=7
  beta (radians) : Outport  Port=8
  gamma (radians) : Outport  Port=9
  wires:
  Vicon Measurements1/2(Y (m)) -> Y (m)/1
  PitchBias V (right)/1 -> signal generator a3/8(PitchBias V (right))
  a2/1 -> signal generator a3/9(a2)
  Phase (deg)/1 -> signal generator a3/7(Phase (deg))
  Vicon Measurements1/4(alpha (radians)) -> alpha (radians)/1
  frequency (hz)/1 -> signal generator a3/3(frequency (hz))
  RollBias V/1 -> signal generator a3/6(RollBias V)
  Bias_v/1 -> signal generator a3/2(Bias_v)
  Vicon Measurements1/6(gamma (radians)) -> gamma (radians)/1
  Amplitude/1 -> signal generator a3/4(Amplitude)
  Vicon Measurements1/5(beta (radians)) -> beta (radians)/1
  signal generator a3/3(D2A DriveSignal 2) -> RW signal/1, PCI-6259 DA1/3
  signal generator a3/1(Bias_D2A) -> bias2/1, PCI-6259 DA1/1
  Vicon Measurements1/1(X (m)) -> X (m)/1
  Vicon Measurements1/3(Z (m)) -> Z (m)/1
  In10/1 -> PCI-6259 DA1/4
  PitchBias V (left)/1 -> signal generator a3/5(PitchBias V (left))
  EnableSignal/1 -> signal generator a3/1(EnableSignal)
  signal generator a3/2(D2A DriveSignal 1) -> LW signal/1, PCI-6259 DA1/2

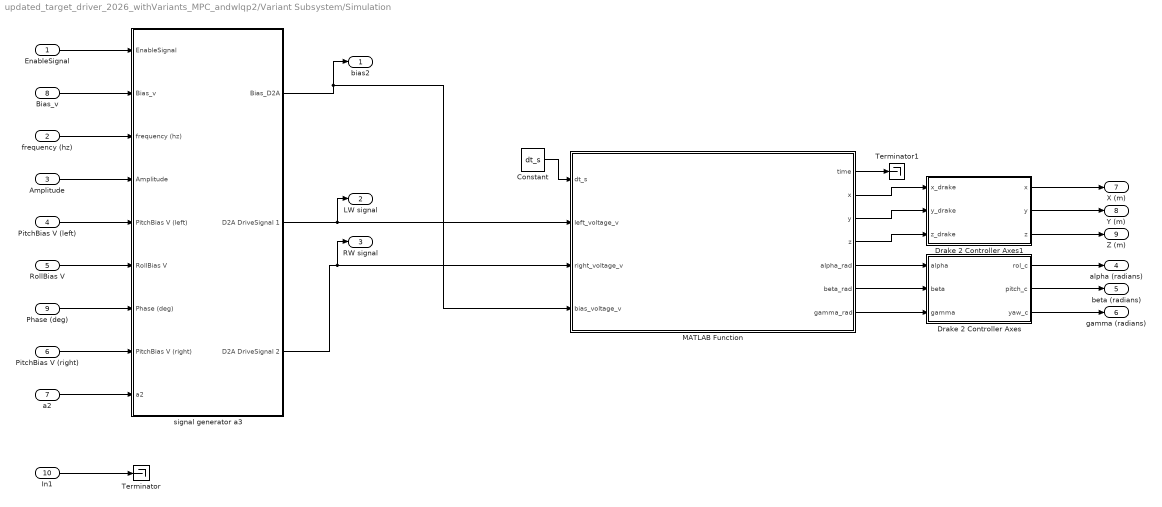
== system updated_target_driver_2026_withVariants_MPC_andwlqp2/Variant Subsystem/Simulation ==
  EnableSignal : Inport
  frequency (hz) : Inport  Port=2
  Amplitude : Inport  Port=3
  PitchBias V (left) : Inport  Port=4
  RollBias V : Inport  Port=5
  PitchBias V (right) : Inport  Port=6
  a2 : Inport  Port=7
  Bias_v : Inport  Port=8
  Phase (deg) : Inport  Port=9
  In1 : Inport  Port=10
  Constant : Constant  Value=dt_s
  Drake 2 Controller Axes : MATLAB Function  TreatAsAtomicUnit=on
  Drake 2 Controller Axes1 : MATLAB Function  TreatAsAtomicUnit=on
  MATLAB Function : MATLAB Function  TreatAsAtomicUnit=on  VariantControl=Choice_1
  Terminator : Terminator
  Terminator1 : Terminator
  signal generator a3 : Subsystem
  bias2 : Outport
  LW signal : Outport  Port=2
  RW signal : Outport  Port=3
  alpha (radians) : Outport  Port=4
  beta (radians) : Outport  Port=5
  gamma (radians) : Outport  Port=6
  X (m) : Outport  Port=7
  Y (m) : Outport  Port=8
  Z (m) : Outport  Port=9
  wires:
  signal generator a3/1(Bias_D2A) -> bias2/1, MATLAB Function/4(bias_voltage_v)
  Constant/1 -> MATLAB Function/1(dt_s)
  signal generator a3/3(D2A DriveSignal 2) -> RW signal/1, MATLAB Function/3(right_voltage_v)
  a2/1 -> signal generator a3/9(a2)
  PitchBias V (left)/1 -> signal generator a3/5(PitchBias V (left))
  Amplitude/1 -> signal generator a3/4(Amplitude)
  Bias_v/1 -> signal generator a3/2(Bias_v)
  PitchBias V (right)/1 -> signal generator a3/8(PitchBias V (right))
  RollBias V/1 -> signal generator a3/6(RollBias V)
  Phase (deg)/1 -> signal generator a3/7(Phase (deg))
  frequency (hz)/1 -> signal generator a3/3(frequency (hz))
  EnableSignal/1 -> signal generator a3/1(EnableSignal)
  In1/1 -> Terminator/1
  MATLAB Function/1(time) -> Terminator1/1
  MATLAB Function/4(z) -> Drake 2 Controller Axes1/3(z_drake)
  MATLAB Function/3(y) -> Drake 2 Controller Axes1/2(y_drake)
  MATLAB Function/2(x) -> Drake 2 Controller Axes1/1(x_drake)
  MATLAB Function/5(alpha_rad) -> Drake 2 Controller Axes/1(alpha)
  MATLAB Function/6(beta_rad) -> Drake 2 Controller Axes/2(beta)
  MATLAB Function/7(gamma_rad) -> Drake 2 Controller Axes/3(gamma)
  Drake 2 Controller Axes/1(rol_c) -> alpha (radians)/1
  Drake 2 Controller Axes/2(pitch_c) -> beta (radians)/1
  Drake 2 Controller Axes/3(yaw_c) -> gamma (radians)/1
  Drake 2 Controller Axes1/2(y) -> Y (m)/1
  Drake 2 Controller Axes1/1(x) -> X (m)/1
  Drake 2 Controller Axes1/3(z) -> Z (m)/1
  signal generator a3/2(D2A DriveSignal 1) -> MATLAB Function/2(left_voltage_v), LW signal/1

== system updated_target_driver_2026_withVariants_MPC_andwlqp2/Vicon Post Processing1/Raw rotation matrix ==
  alpha : Inport
  beta : Inport  Port=2
  gamma : Inport  Port=3
  Mux : Mux  Inputs=9
  Rotation Matrix : Subsystem
  R : Outport
  wires:
  alpha/1 -> Rotation Matrix/1(alpha)
  beta/1 -> Rotation Matrix/2(beta)
  gamma/1 -> Rotation Matrix/3(gamma)
  Mux/1 -> R/1
  Rotation Matrix/1(R11) -> Mux/1
  Rotation Matrix/2(R12) -> Mux/2
  Rotation Matrix/3(R13) -> Mux/3
  Rotation Matrix/4(R21) -> Mux/4
  Rotation Matrix/5(R22) -> Mux/5
  Rotation Matrix/6(R23) -> Mux/6
  Rotation Matrix/7(R31) -> Mux/7
  Rotation Matrix/8(R32) -> Mux/8
  Rotation Matrix/9(R33) -> Mux/9

== system updated_target_driver_2026_withVariants_MPC_andwlqp2/Vicon Post Processing1/Vicon Validity check ==
  "Rotation Matrix " : Inport
  Compare To Zero2 : simulink/Logic and Bit Operations/Compare To Zero  relop===  OutDataTypeStr=uint8
  Constant : Constant
  Data Type Conversion1 : DataTypeConversion  OutDataTypeStr=double  SaturateOnIntegerOverflow=off  RndMeth=Floor
  Delay : Delay  DelayLength=1  InitialCondition=0
  Delay2 : Delay  DelayLength=1  InitialCondition=0
  MATLAB Function3 : MATLAB Function  TreatAsAtomicUnit=on
  SaturatingRamp : DiscreteIntegrator  gainval=sampling_f  ExternalReset=falling  SampleTime=-1  UpperSaturationLimit=1  LowerSaturationLimit=0  ICPrevOutput=DiscIntNeverNeededParam  ICPrevScaledInput=DiscIntNeverNeededParam
  Variant Subsystem1 : Subsystem  Variant=on
  type conv : DataTypeConversion  OutDataTypeStr=double  SaturateOnIntegerOverflow=off  RndMeth=Floor
  "Vicon Update flag " : Outport
  Vicon Count : Outport  Port=2
  wires:
  Delay/1 -> MATLAB Function3/1(R_prev)
  SaturatingRamp/1 -> Data Type Conversion1/1
  type conv/1 -> SaturatingRamp/2
  Constant/1 -> SaturatingRamp/1
  Compare To Zero2/1 -> type conv/1
  "Rotation Matrix "/1 -> MATLAB Function3/2(R_cur), Delay/1
  Delay2/1 -> Vicon Count/1
  Data Type Conversion1/1 -> "Vicon Update flag "/1, Delay2/1
  MATLAB Function3/1(y) -> Variant Subsystem1/1(In1)
  Variant Subsystem1/1(Out1) -> Compare To Zero2/1

== system updated_target_driver_2026_withVariants_MPC_andwlqp2/Force to voltage/Control Mode/Force_to_Voltage1 ==
  note: Mapping from desired Thrust/Torque to Wing traj to Voltage mapping
      |
      | Patrick Hyun 2021 Apr
  note: a2: second-harmonic coefficient
      | Franklin Ho Jun 2026
  "Thrust_desired " : Inport
  Roll_torque_desired : Inport  Port=2
  Pitch_torque_desired : Inport  Port=3
  Yaw_torque_desired : Inport  Port=4
  A : Constant  Commented=on  Value=A
  Desired_Force_to_Voltage : MATLAB Function  TreatAsAtomicUnit=on
  "Force to Trajectory " : MATLAB Function  Commented=on  TreatAsAtomicUnit=on
  "Trajectory to Voltage Input " : MATLAB Function  Commented=on  TreatAsAtomicUnit=on
  left_mapping : Constant  Commented=on  Value=left_mapping
  left_mapping_F_to_Phi : Constant  Commented=on  Value=left_mapping_F_to_Phi
  params_vec : Constant  Value=params_vec
  right_mapping1 : Constant  Commented=on  Value=right_mapping
  right_mapping_F_to_Phi : Constant  Commented=on  Value=right_mapping_F_to_Phi
  drv_amp : Outport
  drv_pitch_left : Outport  Port=2
  drv_pitch_right : Outport  Port=3
  drv_roll : Outport  Port=4
  a2 : Outport  Port=5
  wires:
  left_mapping/1 -> "Trajectory to Voltage Input "/4(left_mapping)
  right_mapping1/1 -> "Trajectory to Voltage Input "/5(right_mapping)
  A/1 -> "Force to Trajectory "/6(A)
  "Force to Trajectory "/1(Phi_left_p2p_desired) -> "Trajectory to Voltage Input "/1(Phi_left_p2p_command)
  "Force to Trajectory "/2(Phi_right_p2p_desired) -> "Trajectory to Voltage Input "/2(Phi_right_p2p_command)
  "Force to Trajectory "/3(Phi_pitch_desired) -> "Trajectory to Voltage Input "/3(Phi_pitch_command)
  left_mapping_F_to_Phi/1 -> "Force to Trajectory "/4(left_mapping_F_to_Phi)
  right_mapping_F_to_Phi/1 -> "Force to Trajectory "/5(right_mapping_F_to_Phi)
  Desired_Force_to_Voltage/4(drv_pitch_right) -> drv_pitch_right/1
  Desired_Force_to_Voltage/3(drv_pitch_left) -> drv_pitch_left/1
  Desired_Force_to_Voltage/2(drv_roll) -> drv_roll/1
  Desired_Force_to_Voltage/1(drv_amp) -> drv_amp/1
  "Thrust_desired "/1 -> Desired_Force_to_Voltage/1(Thrust_desired)
  Pitch_torque_desired/1 -> Desired_Force_to_Voltage/3(Pitch_torque_desired)
  Yaw_torque_desired/1 -> Desired_Force_to_Voltage/4(Yaw_torque_desired)
  params_vec/1 -> Desired_Force_to_Voltage/5(params_vec)
  Desired_Force_to_Voltage/5(a2_coeff) -> a2/1
  Roll_torque_desired/1 -> Desired_Force_to_Voltage/2(Roll_torque_desired)

== system updated_target_driver_2026_withVariants_MPC_andwlqp2/Force to voltage/Replay Mode/Force_to_Voltage1 ==
  note: a2: second-harmonic coefficient
      | Franklin Ho Jun 2026
  note: Mapping from desired Thrust/Torque to Wing traj to Voltage mapping
      |
      | Patrick Hyun 2021 Apr
  "Thrust_desired " : Inport
  Roll_torque_desired : Inport  Port=2
  Pitch_torque_desired : Inport  Port=3
  Yaw_torque_desired : Inport  Port=4
  A : Constant  Commented=on  Value=A
  Desired_Force_to_Voltage : MATLAB Function  TreatAsAtomicUnit=on
  "Force to Trajectory " : MATLAB Function  Commented=on  TreatAsAtomicUnit=on
  Saturation : Saturate  UpperLimit=a2_ub  LowerLimit=a2_lb
  "Trajectory to Voltage Input " : MATLAB Function  Commented=on  TreatAsAtomicUnit=on
  left_mapping : Constant  Commented=on  Value=left_mapping
  left_mapping_F_to_Phi : Constant  Commented=on  Value=left_mapping_F_to_Phi
  params_vec : Constant  Value=params_vec
  right_mapping1 : Constant  Commented=on  Value=right_mapping
  right_mapping_F_to_Phi : Constant  Commented=on  Value=right_mapping_F_to_Phi
  drv_amp : Outport
  drv_pitch_left : Outport  Port=2
  drv_pitch_right : Outport  Port=3
  drv_roll : Outport  Port=4
  a2 : Outport  Port=5
  wires:
  Roll_torque_desired/1 -> Desired_Force_to_Voltage/2(Roll_torque_desired)
  Saturation/1 -> a2/1
  Desired_Force_to_Voltage/5(a2_coeff) -> Saturation/1
  params_vec/1 -> Desired_Force_to_Voltage/5(params_vec)
  Yaw_torque_desired/1 -> Desired_Force_to_Voltage/4(Yaw_torque_desired)
  Pitch_torque_desired/1 -> Desired_Force_to_Voltage/3(Pitch_torque_desired)
  "Thrust_desired "/1 -> Desired_Force_to_Voltage/1(Thrust_desired)
  Desired_Force_to_Voltage/1(drv_amp) -> drv_amp/1
  Desired_Force_to_Voltage/2(drv_roll) -> drv_roll/1
  Desired_Force_to_Voltage/3(drv_pitch_left) -> drv_pitch_left/1
  Desired_Force_to_Voltage/4(drv_pitch_right) -> drv_pitch_right/1
  right_mapping_F_to_Phi/1 -> "Force to Trajectory "/5(right_mapping_F_to_Phi)
  left_mapping_F_to_Phi/1 -> "Force to Trajectory "/4(left_mapping_F_to_Phi)
  "Force to Trajectory "/3(Phi_pitch_desired) -> "Trajectory to Voltage Input "/3(Phi_pitch_command)
  "Force to Trajectory "/2(Phi_right_p2p_desired) -> "Trajectory to Voltage Input "/2(Phi_right_p2p_command)
  "Force to Trajectory "/1(Phi_left_p2p_desired) -> "Trajectory to Voltage Input "/1(Phi_left_p2p_command)
  A/1 -> "Force to Trajectory "/6(A)
  right_mapping1/1 -> "Trajectory to Voltage Input "/5(right_mapping)
  left_mapping/1 -> "Trajectory to Voltage Input "/4(left_mapping)

== system updated_target_driver_2026_withVariants_MPC_andwlqp2/Observer for averaged system1/Attitude Observer/Geometric Averaging Rotation Matix ==
  note: Geometric mean in SO(3)
      | 1) Output the Geometric average over one cycle (n=4 samples: 500Hz vicon sampling and 160Hz flapping signal)
      |
      | Patrick 2021 Mar
  Vicon Update flag : Inport
  Current Rotation : Inport  Port=2
  Averaged quaternion : MATLAB Function  TreatAsAtomicUnit=on
  Delay6 : Delay  DelayLength=1  InitialCondition=0
  Demux3 : Demux
  Demux4 : Demux
  Geometric Averaging Rotation M : Subsystem
  Mux3 : Mux
  Mux4 : Mux
  Raw quaternion : MATLAB Function  TreatAsAtomicUnit=on
  Averaged quaternion output : Outport
  "Averaged Rotation Matrix " : Outport  Port=2
  "Raw quaternion output " : Outport  Port=3
  Previous Averaged Rotation Matrix : Outport  Port=4
  wires:
  Raw quaternion/1(quat) -> Demux4/1
  Demux4/3 -> Mux4/3
  Demux4/4 -> Mux4/4
  Demux4/1 -> Mux4/1
  Demux4/2 -> Mux4/2
  Mux4/1 -> "Raw quaternion output "/1
  Vicon Update flag/1 -> Geometric Averaging Rotation M/2(Vicon Update)
  Current Rotation/1 -> Raw quaternion/1(R), Geometric Averaging Rotation M/1("Current Rotation ")
  Mux3/1 -> Averaged quaternion output/1
  Demux3/4 -> Mux3/4
  Averaged quaternion/1(quat) -> Demux3/1
  Demux3/3 -> Mux3/3
  Geometric Averaging Rotation M/1(Averaged Rotation Matrix) -> Delay6/1, Averaged quaternion/1(R), "Averaged Rotation Matrix "/1
  Demux3/2 -> Mux3/2
  Demux3/1 -> Mux3/1
  Delay6/1 -> Geometric Averaging Rotation M/3("Previous Averaged Rotation "), Previous Averaged Rotation Matrix/1
